simulink model "RC_TOP_and_BOT"  (Simulink 9.2)
settings: Solver=ode1  StartTime=0.0  StopTime=300000.0  FixedStep=0.1  RelTol=1e-3  EnableMultiTasking=on
settings Model: Creator=user  LastModifiedBy=user
settings DataIOCC: SignalLoggingSaveFormat=Dataset
settings DebuggingCC: UnderspecifiedInitializationDetection=Simplified  MergeDetectMultiDrivingBlocksExec=error  SolverPrmCheckMsg=warning  FcnCallInpInsideContextMsg=error  StateNameClashWarn=none
settings GRTTargetCC: CombineOutputUpdateFcns=on  GRTInterface=off
settings ConfigComp: CovSFcnEnable=off

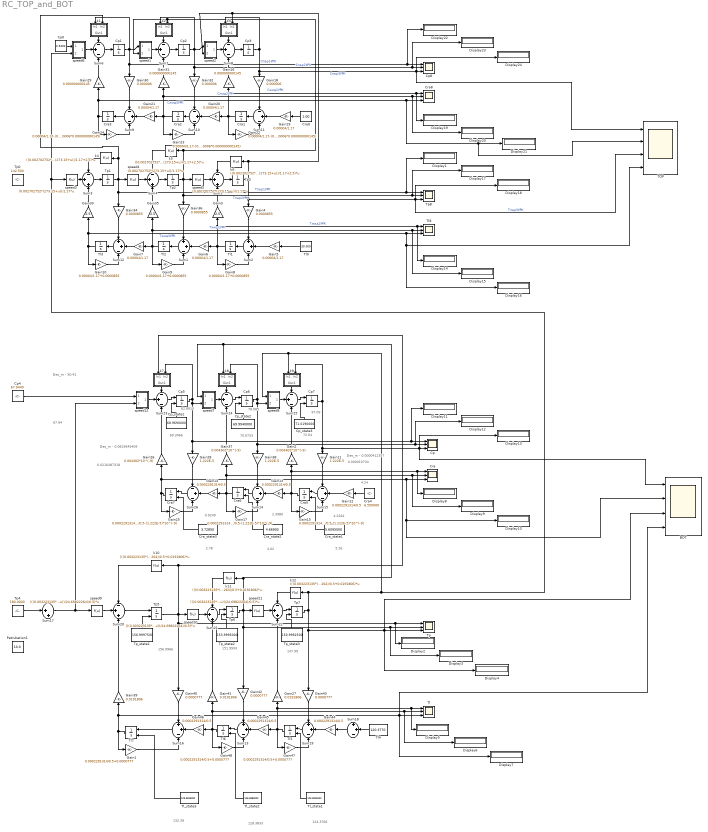
== system RC_TOP_and_BOT ==
  note: Des_m - 0.0000412357
  note: Des_m - 0.0815645409
  note: 0.000010734
  note: 0.0216487318
  note: 0.9249
  note: 2.3980
  note: 4.2264
  note: 62.8910
  note: 78.085
  note: 97.09
  note: 67.94
  note: 2.78
  note: 4.02
  note: 5.26
  note: 72.04
  note: 70.6733
  note: 69.3066
  note: 132.39
  note: 128.3833
  note: 124.3766
  note: 147.99
  note: 151.9933
  note: 156.9966
  note: 4.24
  note: Des_m - 50.41
  BOT : Scope  NumInputPorts=4
  Cp : Scope  NumInputPorts=3
  Cp0 : Constant  Value=0.5300
  Cp1 : Integrator  InitialCondition=0.682000
  Cp2 : Integrator  InitialCondition=0.834000
  Cp3 : Integrator  InitialCondition=0.98600
  Cp4 : Constant  Value=67.9440
  Cp5 : Integrator  InitialConditionSource=external  InitialCondition=69.3066
  Cp6 : Integrator  InitialConditionSource=external  InitialCondition=70.6733
  Cp7 : Integrator  InitialConditionSource=external  InitialCondition=72.04
  Cp8 : Scope  NumInputPorts=3
  Cp_state1 : Constant  Value=68.9690000
  Cp_state2 : Constant  Value=69.9940000
  Cp_state3 : Constant  Value=71.0190000
  Cra : Scope  NumInputPorts=3
  Cra0 : Constant  Value=1.00
  Cra1 : Integrator  InitialCondition=0.8882500
  Cra2 : Integrator  InitialCondition=0.7765000
  Cra3 : Integrator  InitialCondition=0.6647500
  Cra4 : Constant  Value=6.550000
  Cra5 : Integrator  InitialConditionSource=external  InitialCondition=5.26
  Cra6 : Integrator  InitialConditionSource=external  InitialCondition=4.02
  Cra7 : Integrator  InitialConditionSource=external  InitialCondition=2.78
  Cra8 : Scope  NumInputPorts=3
  Cra_state1 : Constant  Value=5.6095000
  Cra_state2 : Constant  Value=4.66900
  Cra_state3 : Constant  Value=3.72850
  Display{1..24} (24 alike) : Display
  Gain1 : Gain  Gain=0.0002291314/0.5+0.0000777
  Gain10 : Gain  Gain=0.00004/1.17+0.0000855
  Gain11 : Gain  Gain=1.222E-5
  Gain{12..14,44..46} (6 alike) : Gain  Gain=0.0002291314/0.5
  Gain15 : Gain  Gain=0.0002291314/0.5-(1.222E-5)*10^(-9)
  Gain16 : Gain  Gain=0.000000000145
  Gain17 : Gain  Gain=0.0002291314/0.5-(1.222E-5)*10^(-9)
  Gain18 : Gain  Gain=0.000006
  Gain{5..7,19..21} (6 alike) : Gain  Gain=0.00004/1.17
  Gain2 : Gain  Gain=0.004302*10^(-9)
  Gain22 : Gain  Gain=0.00004/1.17-(0.000006*0.000000000145)
  Gain23 : Gain  Gain=0.00004/1.17-(0.000006*0.000000000145)
  Gain24 : Gain  Gain=0.00004/1.17-(0.000006*0.000000000145)
  Gain25 : Gain  Gain=0.0002291314/0.5-(1.222E-5)*10^(-9)
  Gain26 : Gain  Gain=0.004302*10^(-9)
  Gain27 : Gain  Gain=0.0191806
  Gain28 : Gain  Gain=1.222E-5
  Gain29 : Gain  Gain=0.000000000145
  Gain3 : Gain  Gain=2.5
  Gain30 : Gain  Gain=0.000006
  Gain31 : Gain  Gain=0.000000000145
  Gain32 : Gain  Gain=0.000006
  Gain33 : Gain  Gain=2.5
  Gain34 : Gain  Gain=0.0000855
  Gain35 : Gain  Gain=2.5
  Gain36 : Gain  Gain=0.0000855
  Gain37 : Gain  Gain=0.004302*10^(-9)
  Gain38 : Gain  Gain=1.222E-5
  Gain39 : Gain  Gain=0.0191806
  Gain4 : Gain  Gain=0.0000855
  Gain40 : Gain  Gain=0.0000777
  Gain41 : Gain  Gain=0.0191806
  Gain42 : Gain  Gain=0.0000777
  Gain43 : Gain  Gain=0.0000777
  Gain47 : Gain  Gain=0.0002291314/0.5+0.0000777
  Gain48 : Gain  Gain=0.0002291314/0.5+0.0000777
  Gain8 : Gain  Gain=0.00004/1.17+0.0000855
  Gain9 : Gain  Gain=0.00004/1.17+0.0000855
  Petrubation1 : Constant  Value=10.0
  Sum{1..2,12..13,16,18..19} (7 alike) : Sum  Inputs=++-
  Sum{6..11,14..15,23..26} (12 alike) : Sum  Inputs=-+-
  Sum17 : Sum  Inputs=|++
  Sum{3..5,20..22} (6 alike) : Sum  Inputs=-++
  TOP : Scope  NumInputPorts=4
  Tl : Scope  NumInputPorts=3
  Tl0 : Constant  Value=30.000
  Tl1 : Integrator  InitialCondition=57.25000
  Tl2 : Integrator  InitialCondition=84.5000
  Tl3 : Integrator  InitialCondition=111.7500
  Tl4 : Constant  Value=120.3770
  Tl5 : Integrator  InitialConditionSource=external  InitialCondition=124.3766
  Tl6 : Integrator  InitialConditionSource=external  InitialCondition=128.3833
  Tl7 : Integrator  InitialConditionSource=external  InitialCondition=132.39
  Tl8 : Scope  NumInputPorts=3
  "Tl_state1 " : Constant  Value=123.3825000
  Tl_state2 : Constant  Value=126.3880000
  Tl_state3 : Constant  Value=129.3935000
  Tp : Scope  NumInputPorts=3
  Tp0 : Constant  Value=142.500
  Tp1 : Integrator  InitialCondition=118.2000
  Tp2 : Integrator  InitialCondition=93.9000
  Tp3 : Integrator  InitialCondition=69.600  IgnoreLimit=on
  Tp4 : Constant  Value=180.0000
  Tp5 : Integrator  InitialConditionSource=external  InitialCondition=156.9966
  Tp6 : Integrator  InitialConditionSource=external  InitialCondition=151.9933
  Tp7 : Integrator  InitialConditionSource=external  InitialCondition=147.99  IgnoreLimit=on
  Tp8 : Scope  NumInputPorts=3
  Tp_state1 : Constant  Value=156.9997500
  Tp_state2 : Constant  Value=153.9995000
  Tp_state3 : Constant  Value=150.9992500
  k1 : Subsystem
  k10 : Fcn  Expr=(((0.003223135*(273+u))/24.69822264)/0.5+0.0191806)*u
  k11 : Fcn  Expr=(((0.003223135*(273+u))/24.69822264)/0.5+0.0191806)*u
  k12 : Fcn  Expr=(((0.003223135*(273+u))/24.69822264)/0.5+0.0191806)*u
  k2 : Subsystem
  k3 : Subsystem
  k4 : Fcn  Expr=((0.002702752*(273.15+u))/1.17+2.5)*u
  k5 : Fcn  Expr=((0.002702752*(273.15+u))/1.17+2.5)*u
  k6 : Fcn  Expr=((0.002702752*(273.15+u))/1.17+2.5)*u
  k7 : Subsystem
  k8 : Subsystem
  k9 : Subsystem
  speed1 : Subsystem
  speed10 : Fcn  Expr=(((0.003223135*(273+u))/24.69822264)/0.5)*u
  speed11 : Fcn  Expr=(((0.003223135*(273+u))/24.69822264)/0.5)*u
  speed12 : Subsystem
  speed2 : Subsystem
  speed3 : Fcn  Expr=(0.002702752*(273.15+u))/1.17*u
  speed4 : Fcn  Expr=(0.002702752*(273.15+u))/1.17*u
  speed5 : Fcn  Expr=(0.002702752*(273.15+u))/1.17*u
  speed6 : Subsystem
  speed7 : Subsystem
  speed8 : Subsystem
  speed9 : Fcn  Expr=(((0.003223135*(273+u))/24.69822264)/0.5)*u
  wires:
  Sum6/1 -> Cp1/1
  speed1/1(Out1) -> Sum7/2
  Sum7/1 -> Cp2/1
  speed2/1(Out1) -> Sum8/2
  Sum8/1 -> Cp3/1
  Cp1/1 -> Cp8/1, Display22/1, Gain30/1, k1/1(In1), speed1/1(In1)  "Cпар1УРК"
  Cp2/1 -> Display23/1, Cp8/2, Gain32/1, speed2/1(In1), k2/1(In1)  "Cпар2УРК"
  Gain29/1 -> Sum6/3
  Cp3/1 -> TOP/1, Cp8/3, Display24/1, Gain18/1, k3/1(In1)  "Cпар3УРК"
  Gain31/1 -> Sum7/3
  Gain16/1 -> Sum8/3
  Gain30/1 -> Sum9/1
  Gain32/1 -> Sum10/1
  Gain18/1 -> Sum11/1
  Gain19/1 -> Sum11/2
  Sum11/1 -> Cra1/1
  Cra1/1 -> Gain22/1, Gain20/1, Display19/1, Cra8/1, Gain16/1  "Cжид1УРК"
  Gain20/1 -> Sum10/2
  Sum10/1 -> Cra2/1
  Cra2/1 -> Gain23/1, Gain21/1, Display20/1, Cra8/2, Gain31/1  "Cжид2УРК"
  Gain21/1 -> Sum9/2
  Sum9/1 -> Cra3/1
  Cra3/1 -> Gain24/1, TOP/2, Display21/1, Cra8/3, Gain29/1  "Cжид3УРК"
  Gain22/1 -> Sum11/3
  Gain23/1 -> Sum10/3
  Gain24/1 -> Sum9/3
  speed3/1 -> Sum3/2
  k4/1 -> Sum3/1
  Sum3/1 -> Tp1/1
  speed4/1 -> Sum4/2
  k5/1 -> Sum4/1
  Sum4/1 -> Tp2/1
  speed5/1 -> Sum5/2
  k6/1 -> Sum5/1
  Sum5/1 -> Tp3/1
  Tp1/1 -> Display1/1, Tp8/1, Gain34/1, k4/1, k1/2(In2), speed4/1  "Tпар1УРК"
  Gain33/1 -> Sum3/3
  Tp3/1 -> TOP/3, Display18/1, Tp8/3, Gain4/1, k6/1, k3/2(In2), speed2/2(In2)  "Tпар3УРК"
  Gain35/1 -> Sum4/3
  Gain3/1 -> Sum5/3
  Gain34/1 -> Sum12/1
  Gain36/1 -> Sum1/1
  Gain4/1 -> Sum2/1
  Gain5/1 -> Sum2/2
  Sum2/1 -> Tl1/1
  Tl1/1 -> Gain8/1, Gain6/1, Tl8/1, Display14/1, Gain3/1  "Tжид1УРК"
  Gain6/1 -> Sum1/2
  Sum1/1 -> Tl2/1
  Tl2/1 -> Gain9/1, Gain7/1, Tl8/2, Display15/1, Gain35/1  "Tжид2УРК"
  Gain7/1 -> Sum12/2
  Sum12/1 -> Tl3/1
  Tl3/1 -> Gain10/1, TOP/4, Display16/1, Tl8/3, Gain33/1  "Tжид3УРК"
  Gain8/1 -> Sum2/3
  Gain9/1 -> Sum1/3
  Gain10/1 -> Sum12/3
  speed6/1(Out1) -> Sum6/2
  Cp0/1 -> speed6/1(In1)
  k1/1(Out1) -> Sum6/1
  k2/1(Out1) -> Sum7/1
  k3/1(Out1) -> Sum8/1
  Cra0/1 -> Gain19/1
  Tl0/1 -> Gain5/1
  Sum23/1 -> Cp5/1
  speed7/1(Out1) -> Sum24/2
  Sum24/1 -> Cp6/1
  speed8/1(Out1) -> Sum25/2
  Sum25/1 -> Cp7/1
  Cp5/1 -> speed7/2(In2), Gain28/1, Cp/1, Display11/1, k7/2(In2)
  Gain26/1 -> Sum23/3
  Cp7/1 -> k9/2(In2), Gain11/1, BOT/1, Display13/1, Cp/3
  Gain37/1 -> Sum24/3
  Gain2/1 -> Sum25/3
  Gain28/1 -> Sum26/1
  Gain38/1 -> Sum14/1
  Gain11/1 -> Sum15/1
  Gain12/1 -> Sum15/2
  Sum15/1 -> Cra5/1
  Cra5/1 -> Gain15/1, Gain13/1, Gain2/1, Display8/1, Cra/1
  Gain13/1 -> Sum14/2
  Sum14/1 -> Cra6/1
  Gain14/1 -> Sum26/2
  Sum26/1 -> Cra7/1
  Gain15/1 -> Sum15/3
  Gain17/1 -> Sum14/3
  Gain25/1 -> Sum26/3
  speed9/1 -> Sum20/2
  k10/1 -> Sum20/1
  Sum20/1 -> Tp5/1
  speed10/1 -> Sum21/2
  k11/1 -> Sum21/1
  Sum21/1 -> Tp6/1
  speed11/1 -> Sum22/2
  k12/1 -> Sum22/1
  Sum22/1 -> Tp7/1
  Gain39/1 -> Sum20/3
  Gain41/1 -> Sum21/3
  Gain27/1 -> Sum22/3
  Gain40/1 -> Sum16/1
  Gain42/1 -> Sum13/1
  Gain43/1 -> Sum19/1
  Gain44/1 -> Sum19/2
  Sum19/1 -> Tl5/1
  Tl5/1 -> Gain47/1, Gain45/1, Gain27/1, Display5/1, Tl/1
  Gain45/1 -> Sum13/2
  Sum13/1 -> Tl6/1
  Gain46/1 -> Sum16/2
  Sum16/1 -> Tl7/1
  Gain47/1 -> Sum19/3
  Gain48/1 -> Sum13/3
  Gain1/1 -> Sum16/3
  speed12/1(Out1) -> Sum23/2
  Cp4/1 -> speed12/1(In1)
  k7/1(Out1) -> Sum23/1
  k8/1(Out1) -> Sum24/1
  k9/1(Out1) -> Sum25/1
  Cra4/1 -> Gain12/1
  Sum17/1 -> speed9/1, speed12/2(In2)
  Sum18/1 -> Gain44/1
  Tp4/1 -> Sum17/1
  Tl4/1 -> Sum18/2
  Tp6/1 -> Gain42/1, Display3/1, Tp/2, k11/1, speed7/1(In1), k8/1(In1), speed11/1
  Tp_state1/1 -> Tp5/2
  Tp_state3/1 -> Tp7/2
  "Tl_state1 "/1 -> Tl5/2
  Tl_state2/1 -> Tl6/2
  Tl_state3/1 -> Tl7/2
  Cp_state1/1 -> Cp5/2
  Cp_state2/1 -> Cp6/2
  Cp_state3/1 -> Cp7/2
  Cra_state1/1 -> Cra5/2
  Cra_state2/1 -> Cra6/2
  Cra_state3/1 -> Cra7/2
  Tp_state2/1 -> Tp6/2
  Tp7/1 -> Gain43/1, BOT/3, Display4/1, Tp/3, k12/1, k9/1(In1), speed8/1(In1), speed6/2(In2), speed3/1
  Tp2/1 -> Display17/1, Tp8/2, Gain36/1, k5/1, speed1/2(In2), k2/2(In2), speed5/1  "Tпар2УРК"
  Tl6/1 -> Gain48/1, Gain46/1, Gain41/1, Display6/1, Tl/2
  Cra6/1 -> Gain17/1, Gain14/1, Gain37/1, Display9/1, Cra/2
  Cp6/1 -> speed8/2(In2), Gain38/1, Display12/1, Cp/2, k8/2(In2)
  Tp5/1 -> Gain40/1, Display2/1, Tp/1, k10/1, k7/1(In1), speed10/1
  Tl7/1 -> Gain1/1, Gain39/1, BOT/4, Display7/1, Tl/3
  Cra7/1 -> Gain25/1, Gain26/1, BOT/2, Display10/1, Cra/3

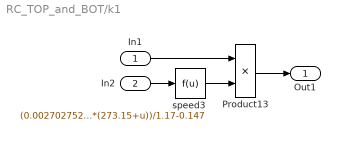
== system RC_TOP_and_BOT/k1 ==
  In1 : Inport
  In2 : Inport  Port=2
  Product13 : Product  SaturateOnIntegerOverflow=on  InputSameDT=on  OutDataTypeStr=Inherit: Same as first input
  speed3 : Fcn  Expr=(0.002702752*(273.15+u))/1.17-0.147
  Out1 : Outport
  wires:
  Product13/1 -> Out1/1
  speed3/1 -> Product13/2
  In2/1 -> speed3/1
  In1/1 -> Product13/1

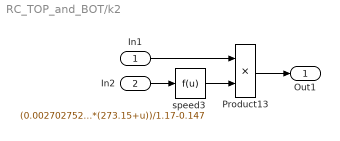
== system RC_TOP_and_BOT/k2 ==
  In1 : Inport
  In2 : Inport  Port=2
  Product13 : Product  SaturateOnIntegerOverflow=on  InputSameDT=on  OutDataTypeStr=Inherit: Same as first input
  speed3 : Fcn  Expr=(0.002702752*(273.15+u))/1.17-0.147
  Out1 : Outport
  wires:
  In1/1 -> Product13/1
  In2/1 -> speed3/1
  speed3/1 -> Product13/2
  Product13/1 -> Out1/1

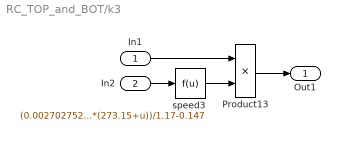
== system RC_TOP_and_BOT/k3 ==
  In1 : Inport
  In2 : Inport  Port=2
  Product13 : Product  SaturateOnIntegerOverflow=on  InputSameDT=on  OutDataTypeStr=Inherit: Same as first input
  speed3 : Fcn  Expr=(0.002702752*(273.15+u))/1.17-0.147
  Out1 : Outport
  wires:
  Product13/1 -> Out1/1
  speed3/1 -> Product13/2
  In2/1 -> speed3/1
  In1/1 -> Product13/1

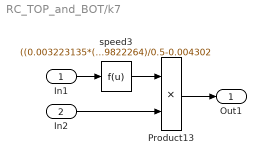
== system RC_TOP_and_BOT/k7 ==
  In1 : Inport
  In2 : Inport  Port=2
  Product13 : Product  SaturateOnIntegerOverflow=on  InputSameDT=on  OutDataTypeStr=Inherit: Same as first input
  speed3 : Fcn  Expr=((0.003223135*(273+u))/24.69822264)/0.5-0.004302
  Out1 : Outport
  wires:
  Product13/1 -> Out1/1
  speed3/1 -> Product13/1
  In1/1 -> speed3/1
  In2/1 -> Product13/2

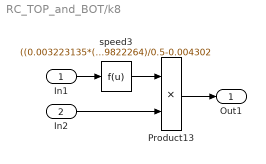
== system RC_TOP_and_BOT/k8 ==
  In1 : Inport
  In2 : Inport  Port=2
  Product13 : Product  SaturateOnIntegerOverflow=on  InputSameDT=on  OutDataTypeStr=Inherit: Same as first input
  speed3 : Fcn  Expr=((0.003223135*(273+u))/24.69822264)/0.5-0.004302
  Out1 : Outport
  wires:
  Product13/1 -> Out1/1
  speed3/1 -> Product13/1
  In1/1 -> speed3/1
  In2/1 -> Product13/2

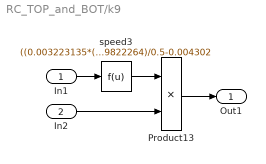
== system RC_TOP_and_BOT/k9 ==
  In1 : Inport
  In2 : Inport  Port=2
  Product13 : Product  SaturateOnIntegerOverflow=on  InputSameDT=on  OutDataTypeStr=Inherit: Same as first input
  speed3 : Fcn  Expr=((0.003223135*(273+u))/24.69822264)/0.5-0.004302
  Out1 : Outport
  wires:
  Product13/1 -> Out1/1
  speed3/1 -> Product13/1
  In1/1 -> speed3/1
  In2/1 -> Product13/2

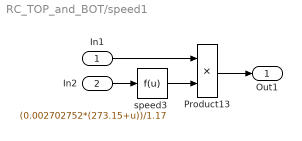
== system RC_TOP_and_BOT/speed1 ==
  In1 : Inport
  In2 : Inport  Port=2
  Product13 : Product  SaturateOnIntegerOverflow=on  InputSameDT=on  OutDataTypeStr=Inherit: Same as first input
  speed3 : Fcn  Expr=(0.002702752*(273.15+u))/1.17
  Out1 : Outport
  wires:
  Product13/1 -> Out1/1
  speed3/1 -> Product13/2
  In2/1 -> speed3/1
  In1/1 -> Product13/1

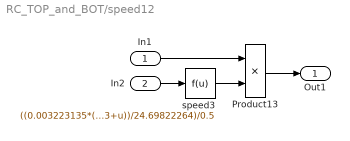
== system RC_TOP_and_BOT/speed12 ==
  In1 : Inport
  In2 : Inport  Port=2
  Product13 : Product  SaturateOnIntegerOverflow=on  InputSameDT=on  OutDataTypeStr=Inherit: Same as first input
  speed3 : Fcn  Expr=((0.003223135*(273+u))/24.69822264)/0.5
  Out1 : Outport
  wires:
  In1/1 -> Product13/1
  In2/1 -> speed3/1
  speed3/1 -> Product13/2
  Product13/1 -> Out1/1

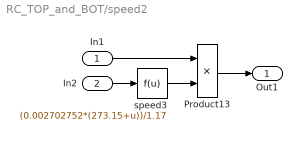
== system RC_TOP_and_BOT/speed2 ==
  In1 : Inport
  In2 : Inport  Port=2
  Product13 : Product  SaturateOnIntegerOverflow=on  InputSameDT=on  OutDataTypeStr=Inherit: Same as first input
  speed3 : Fcn  Expr=(0.002702752*(273.15+u))/1.17
  Out1 : Outport
  wires:
  In1/1 -> Product13/1
  In2/1 -> speed3/1
  speed3/1 -> Product13/2
  Product13/1 -> Out1/1

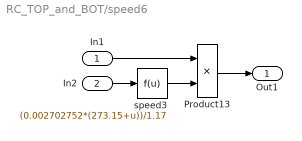
== system RC_TOP_and_BOT/speed6 ==
  In1 : Inport
  In2 : Inport  Port=2
  Product13 : Product  SaturateOnIntegerOverflow=on  InputSameDT=on  OutDataTypeStr=Inherit: Same as first input
  speed3 : Fcn  Expr=(0.002702752*(273.15+u))/1.17
  Out1 : Outport
  wires:
  In1/1 -> Product13/1
  In2/1 -> speed3/1
  speed3/1 -> Product13/2
  Product13/1 -> Out1/1

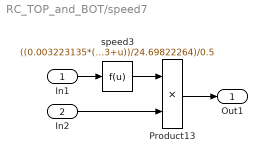
== system RC_TOP_and_BOT/speed7 ==
  In1 : Inport
  In2 : Inport  Port=2
  Product13 : Product  SaturateOnIntegerOverflow=on  InputSameDT=on  OutDataTypeStr=Inherit: Same as first input
  speed3 : Fcn  Expr=((0.003223135*(273+u))/24.69822264)/0.5
  Out1 : Outport
  wires:
  Product13/1 -> Out1/1
  In2/1 -> Product13/2
  speed3/1 -> Product13/1
  In1/1 -> speed3/1

== system RC_TOP_and_BOT/speed8 ==
  In1 : Inport
  In2 : Inport  Port=2
  Product13 : Product  SaturateOnIntegerOverflow=on  InputSameDT=on  OutDataTypeStr=Inherit: Same as first input
  speed3 : Fcn  Expr=((0.003223135*(273+u))/24.69822264)/0.5
  Out1 : Outport
  wires:
  Product13/1 -> Out1/1
  In2/1 -> Product13/2
  speed3/1 -> Product13/1
  In1/1 -> speed3/1
